simulink model "MI6FS_HE_6PhS"  (R2023a)
settings: Solver=FixedStepAuto  StartTime=0  StopTime=L  FixedStep=Ts  RelTol=1e-3
values from neighbouring files (symbols this model uses):
  A = exp(j*pi/3)    [Parameters.m]
  deg = 0    [Parameters.m]
  FV = 9.8    [Parameters.m]
  J = 0.0243    [Parameters.m]
  Lrr = [((1/3*Lm)+Llr) 1/6*Lm -1/6*Lm -1/3*Lm -1/6*Lm 1/6*Lm;        1/6*Lm ((1/3*Lm)+Llr) 1/6*Lm -1/6*Lm -1/3*Lm -1/6*Lm;        -1/6*Lm 1/6*Lm ((1/3*Lm)+Llr) 1/6*Lm -1/6*Lm -1/3*Lm;        -1/3*Lm -1/6*Lm 1/6*Lm ((1/3*Lm)+Llr) 1/6*Lm -1/6*Lm;        -1/6*Lm -1/3*Lm -1/6*Lm 1/6*Lm ((1/3*Lm)+Llr) 1/6*Lm;        1/6*Lm -1/6*Lm -1/3*Lm -1/6*Lm 1/6*Lm ((1/3*Lm)+Llr)]    [Parameters.m]
  Lrs = transpose(Lsr)    [Parameters.m]
  Lsr = [0 (pi/3) 2*(pi/3) 3*(pi/3) 4*(pi/3) 5*(pi/3);        -(pi/3) 0 (pi/3) 2*(pi/3) 3*(pi/3) 4*(pi/3);        -2*(pi/3) -(pi/3) 0 (pi/3) 2*(pi/3) 3*(pi/3);        -3*(pi/3) -2*(pi/3) -(pi/3) 0 (pi/3) 2*(pi/3);        -4*(pi/3) -3*(pi/3) -2*(pi/3) -(pi/3) 0 (pi/3);        -5*(pi/3) -4*(pi/3) -3*(pi/3) -2*(pi/3) -(pi/3) 0]    [Parameters.m]
  Lss = [((1/3*Lm)+Lls) 1/6*Lm -1/6*Lm -1/3*Lm -1/6*Lm 1/6*Lm;        1/6*Lm ((1/3*Lm)+Lls) 1/6*Lm -1/6*Lm -1/3*Lm -1/6*Lm;        -1/6*Lm 1/6*Lm ((1/3*Lm)+Lls) 1/6*Lm -1/6*Lm -1/3*Lm;        -1/3*Lm -1/6*Lm 1/6*Lm ((1/3*Lm)+Lls) 1/6*Lm -1/6*Lm;        -1/6*Lm -1/3*Lm -1/6*Lm 1/6*Lm ((1/3*Lm)+Lls) 1/6*Lm;        1/6*Lm -1/6*Lm -1/3*Lm -1/6*Lm 1/6*Lm ((1/3*Lm)+Lls)]    [Parameters.m]
  Lto = 0    [Parameters.m]
  Msr = (1/3)*Lm    (= 0.0620333333333)    [Parameters.m]
  p = 2    [Parameters.m]
  Rcore = 811    [Parameters.m]
  Rrr = Rr*eye(6,6)    [Parameters.m]
  Rss = Rs*eye(6,6)    [Parameters.m]
  Tav = 0.23    [Parameters.m]
  Ts = 1/Fs    (= 1e-05)    [Parameters.m]
  Us = sqrt(2)*180    [Parameters.m]
undefined symbols (not defined in the file or in its folder): DiscIntNeverNeededParam, j
libraries: spsFourierLib x84, spsVoltageMeasurementLib x13, spsACVoltageSourceLib x6, spsControlledCurrentSourceLib x6, spsCurrentMeasurementLib x6, spsSeriesRLCBranchLib x6, spsSequenceAnalyzerLib x6, sharedutil x5, eeRmsMeasurement x2, eeGeneralControl x1, spsSequenceAnalyzerPhasorLib x1, spsabctoAlphaBetaZeroLib x1
(part 1 of 3)
settings Model: Creator=Hugo  LastModifiedBy=HUGO
settings SolverCC: AlgebraicLoopSolver=TrustRegion
settings DataIOCC: SaveFormat=StructureWithTime  SaveTime=off
settings DebuggingCC: UnconnectedInputMsg=warning  UnconnectedOutputMsg=warning  UnconnectedLineMsg=warning  UnderSpecifiedDimensionMsg=warning
settings ModelReferenceCC: EnableRefExpFcnMdlSchedulingChecks=on
settings SFSimCC: CustomCodeUndefinedFunction=UseInterfaceOnly
settings RTWCC: DLArmComputeVersion=19.05

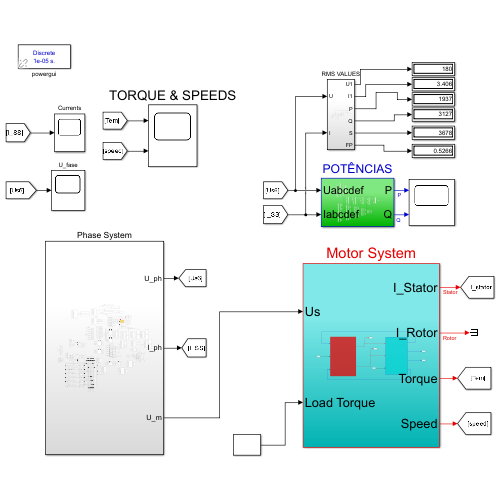
[thumbnail: Simulink's stored preview of the top-level diagram]
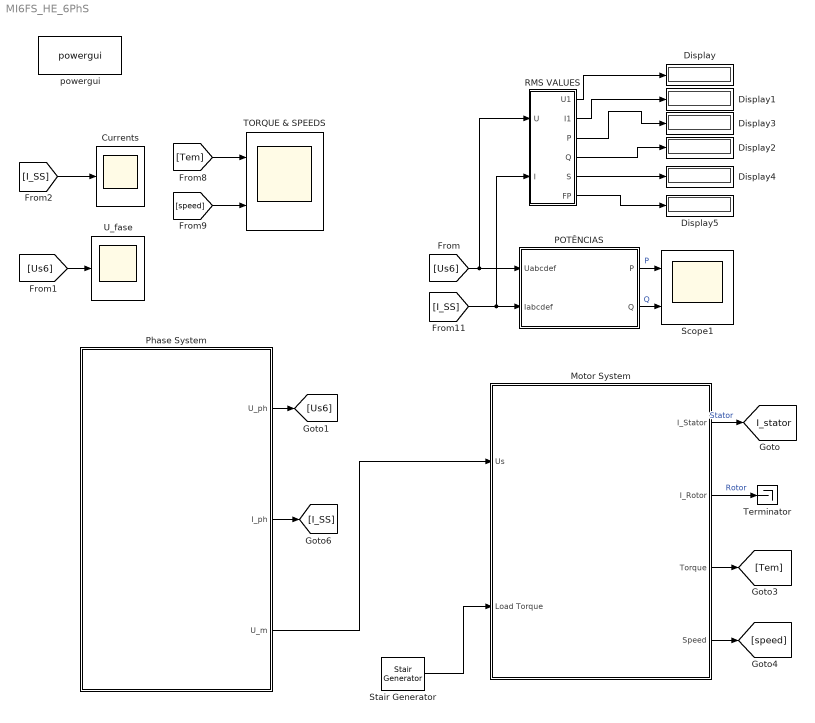
== system MI6FS_HE_6PhS ==
  Currents : Scope
  Display{,1..5} (6 alike) : Display
  Motor System : Subsystem
  POTÊNCIAS : Subsystem
  Phase System : Subsystem
  RMS VALUES : Subsystem
  Scope1 : Scope  NumInputPorts=2
  Stair Generator : spsStairGeneratorLib/Stair Generator  t=[0, 0.5]  e=[0, FV]  Ts=Ts
  TORQUE & SPEEDS : Scope  NumInputPorts=2
  Terminator : Terminator
  U_fase : Scope
  powergui : spspowerguiLib/powergui  Priority=1  SimulationMode=Discrete  SampleTime=Ts  frequency=60  Iterations=50  frequencyindice=50  Pbase=100e6  ErrMax=1e-4  UnitsV=kV  UnitsW=MW  buscounter=0  FunctionMessages=off  echomessages=off  EnableUseOfTLC=off  CurrentSourceSwitches=off  DisableSnubberDevices=off  DisableRonSwitches=off  DisableVfSwitches=off  DisplayEquations=off  AutomaticDiscreteSolvers=off  SolverType=Tustin/Backward Euler (TBE)  Interpol=off  ExternalGateDelay=off  methode=off  Ts=100  x0status=blocks  SPID=on  SwTol=0  HookPort=off  NonlinearTolerance=0  nMaxIteration=15  ContinueOnMaxIteration=off  RestoreLinks=warning  ResistiveCurrentMeasurement=off  Frange=[0:2:500]  Ylog=off  Xlog=on  ShowGrid=off  save=off  variable=ZData  structure=0  ZoomFFT=off  StartTime=0.0  cycles=1  DisplayStyle=1  fundamental=60  FreqAxis=off  MaxFrequency=1000  frequencyindicesteady=1  RmsSteady=1  display=off
  tag scope: I_stator=global
  wires:
  POTÊNCIAS/1(P) -> Scope1/1  "P"
  POTÊNCIAS/2(Q) -> Scope1/2  "Q"
  Motor System/1(I_Stator) -> [I_stator]  "Stator"
  [I_SS] -> POTÊNCIAS/2(Iabcdef), RMS VALUES/2(I)
  Motor System/2(I_Rotor) -> Terminator/1  "Rotor"
  Motor System/3(Torque) -> [Tem]
  Motor System/4(Speed) -> [speed]
  RMS VALUES/1(U1) -> Display/1
  RMS VALUES/2(I1) -> Display1/1
  RMS VALUES/4(Q) -> Display2/1
  RMS VALUES/3(P) -> Display3/1
  RMS VALUES/5(S) -> Display4/1
  RMS VALUES/6(FP) -> Display5/1
  [Us6] -> POTÊNCIAS/1(Uabcdef), RMS VALUES/1(U)
  [Tem] -> TORQUE & SPEEDS/1
  [speed] -> TORQUE & SPEEDS/2
  Phase System/3(U_m) -> Motor System/1(Us)
  Stair Generator/1 -> Motor System/2(Load Torque)
  Phase System/1(U_ph) -> [Us6]
  Phase System/2(I_ph) -> [I_SS]
  [I_SS] -> Currents/1
  [Us6] -> U_fase/1

== system MI6FS_HE_6PhS/Motor System ==
  Us : Inport
  Load Torque : Inport  Port=2
  MECHANICAL SYSTEM : Subsystem
  "MOTOR SYSTEM EQUATIONS " : Subsystem
  I_Stator : Outport  VectorParamsAs1DForOutWhenUnconnected=off
  I_Rotor : Outport  Port=2  VectorParamsAs1DForOutWhenUnconnected=off
  Torque : Outport  Port=3  VectorParamsAs1DForOutWhenUnconnected=off
  Speed : Outport  Port=4  VectorParamsAs1DForOutWhenUnconnected=off
  wires:
  "MOTOR SYSTEM EQUATIONS "/1(I_stator) -> I_Stator/1, MECHANICAL SYSTEM/1(I_s)
  Load Torque/1 -> MECHANICAL SYSTEM/3(TLoad)
  "MOTOR SYSTEM EQUATIONS "/2("I_rotor ") -> MECHANICAL SYSTEM/2(I_r), I_Rotor/1
  Us/1 -> "MOTOR SYSTEM EQUATIONS "/2(Us)
  MECHANICAL SYSTEM/4("Teta_R [rad] ") -> "MOTOR SYSTEM EQUATIONS "/3(Teta_R)
  MECHANICAL SYSTEM/1(We [rads/s]) -> "MOTOR SYSTEM EQUATIONS "/1(We)
  MECHANICAL SYSTEM/2(Tem [Nm]) -> Torque/1
  MECHANICAL SYSTEM/3(n [rpm]) -> Speed/1

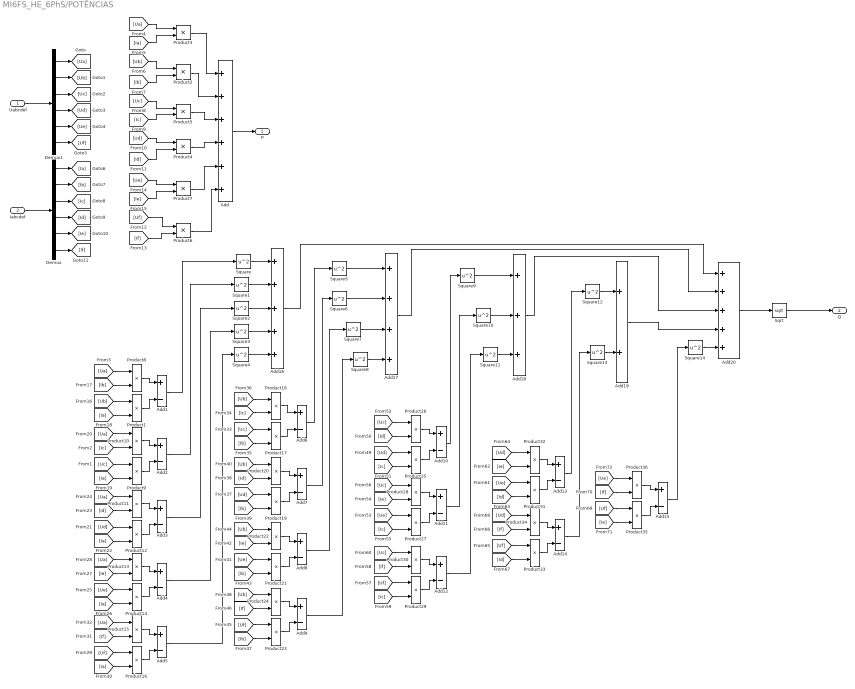
== system MI6FS_HE_6PhS/POTÊNCIAS ==
  Uabcdef : Inport
  Iabcdef : Inport  Port=2
  Add : Sum  Inputs=6
  Add{1..15} (15 alike) : Sum  Inputs=+-
  Add16 : Sum  Inputs=+++++
  Add17 : Sum  Inputs=++++
  Add18 : Sum  Inputs=+++
  Add19 : Sum
  Add20 : Sum  Inputs=5
  Demux : Demux  Outputs=6
  Demux1 : Demux  Outputs=6
  Product{1..36} (36 alike) : Product
  Sqrt : Sqrt
  Square{,1..14} (15 alike) : Math  Operator=square  SignedPower=on
  P : Outport  VectorParamsAs1DForOutWhenUnconnected=off
  Q : Outport  Port=2  VectorParamsAs1DForOutWhenUnconnected=off
  wires:
  Iabcdef/1 -> Demux/1
  Uabcdef/1 -> Demux1/1
  Demux1/1 -> [Ua]
  Demux1/2 -> [Ub]
  Demux1/3 -> [Uc]
  Demux1/4 -> [Ud]
  Demux1/5 -> [Ue]
  Demux1/6 -> [Uf]
  Demux/1 -> [Ia]
  Demux/2 -> [Ib]
  Demux/3 -> [Ic]
  Demux/6 -> [If]
  Demux/4 -> [Id]
  Demux/5 -> [Ie]
  [Ud] -> Product4/1
  [Id] -> Product4/2
  [Ue] -> Product7/1
  [Ie] -> Product7/2
  [Uf] -> Product6/1
  Product2/1 -> Add/2
  Product5/1 -> Add/3
  Product4/1 -> Add/4
  Product7/1 -> Add/5
  Product6/1 -> Add/6
  Product3/1 -> Add/1
  Add/1 -> P/1
  [Ic] -> Product5/2
  [Uc] -> Product5/1
  [Ie] -> Product28/2
  Product17/1 -> Add6/2
  [Id] -> Product33/2
  [If] -> Product30/2
  [Ic] -> Product25/2
  Product32/1 -> Add13/1
  Product30/1 -> Add12/1
  [Ic] -> Product29/2
  [Ia] -> Product9/2
  Product8/1 -> Add1/1
  [Uf] -> Product29/1
  Product15/1 -> Add5/1
  [Id] -> Product26/2
  Product19/1 -> Add7/2
  [Ue] -> Product27/1
  [Ub] -> Product24/1
  [Ud] -> Product25/1
  Product24/1 -> Add9/1
  [Ib] -> Product23/2
  [Uc] -> Product28/1
  Product27/1 -> Add11/2
  Product25/1 -> Add10/2
  [Ib] -> Product21/2
  [Ua] -> Product8/1
  [Ub] -> Product22/1
  [Ue] -> Product21/1
  [Ie] -> Product22/2
  [Uc] -> Product17/1
  Product20/1 -> Add7/1
  Product21/1 -> Add8/2
  [Id] -> Product20/2
  Product18/1 -> Add6/1
  [Ic] -> Product18/2
  Product16/1 -> Add5/2
  [Ua] -> Product10/1
  [Ud] -> Product12/1
  [Ub] -> Product18/1
  [Ib] -> Product8/2
  [If] -> Product15/2
  [Id] -> Product11/2
  Product14/1 -> Add4/2
  [Ue] -> Product14/1
  Product13/1 -> Add4/1
  Product10/1 -> Add2/1
  [Ua] -> Product11/1
  Product11/1 -> Add3/1
  [Ud] -> Product19/1
  [Ub] -> Product1/1
  Add17/1 -> Add20/2
  [Ib] -> Product19/2
  Add6/1 -> Square5/1
  Add15/1 -> Square14/1
  [Uc] -> Product26/1
  Add19/1 -> Add20/4
  Add16/1 -> Add20/1
  Add7/1 -> Square6/1
  [Ia] -> Product16/2
  Product23/1 -> Add9/2
  [Id] -> Product31/2
  [Ie] -> Product13/2
  Add10/1 -> Square9/1
  [Ie] -> Product32/2
  [Ia] -> Product12/2
  Product29/1 -> Add12/2
  [Ue] -> Product31/1
  Product35/1 -> Add15/2
  Product12/1 -> Add3/2
  [Ia] -> Product14/2
  [Ub] -> Product20/1
  Product28/1 -> Add11/1
  Add12/1 -> Square11/1
  Add14/1 -> Square13/1
  Add3/1 -> Square2/1
  Add11/1 -> Square10/1
  [Ic] -> Product10/2
  Add9/1 -> Square8/1
  [Ib] -> Product17/2
  Add13/1 -> Square12/1
  Add18/1 -> Add20/3
  [Ua] -> Product15/1
  Add1/1 -> Square/1
  [Ua] -> Product13/1
  Product36/1 -> Add15/1
  Add4/1 -> Square3/1
  Add2/1 -> Square1/1
  [If] -> Product36/2
  Add5/1 -> Square4/1
  [Uf] -> Product33/1
  [If] -> Product24/2
  Product9/1 -> Add2/2
  Product1/1 -> Add1/2
  [Uc] -> Product9/1
  Add8/1 -> Square7/1
  [Uf] -> Product23/1
  Product22/1 -> Add8/1
  [Uc] -> Product30/1
  Product26/1 -> Add10/1
  [Ud] -> Product32/1
  [Ia] -> Product1/2
  [Uf] -> Product16/1
  Product33/1 -> Add14/2
  [Uf] -> Product35/1
  Product31/1 -> Add13/2
  [Ie] -> Product35/2
  [Ue] -> Product36/1
  [If] -> Product34/2
  [Ic] -> Product27/2
  Product34/1 -> Add14/1
  [Ud] -> Product34/1
  [Ua] -> Product3/1
  [Ub] -> Product2/1
  [If] -> Product6/2
  Sqrt/1 -> Q/1
  Square/1 -> Add16/1
  Square1/1 -> Add16/2
  Square2/1 -> Add16/3
  Square3/1 -> Add16/4
  Square4/1 -> Add16/5
  Square5/1 -> Add17/1
  Square6/1 -> Add17/2
  Square7/1 -> Add17/3
  Square8/1 -> Add17/4
  Square9/1 -> Add18/1
  Square10/1 -> Add18/2
  Square11/1 -> Add18/3
  Square12/1 -> Add19/1
  Square13/1 -> Add19/2
  Square14/1 -> Add20/5
  Add20/1 -> Sqrt/1
  [Ia] -> Product3/2
  [Ib] -> Product2/2

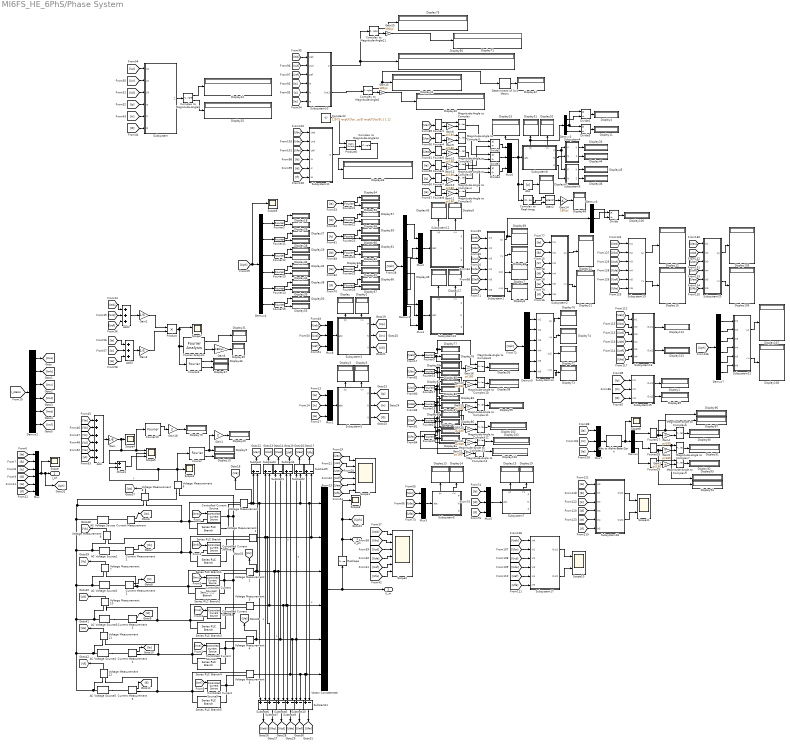
== system MI6FS_HE_6PhS/Phase System ==
  AC Voltage Source : spsACVoltageSourceLib/AC Voltage Source  Amplitude=Us  Phase=deg  Frequency=50  SampleTime=Ts  Measurements=None  BusType=swing  Pref=10e3  Qref=0  Qmin=-inf  Qmax=+inf
  AC Voltage Source1 : spsACVoltageSourceLib/AC Voltage Source  Amplitude=Us  Phase=-60  Frequency=50  SampleTime=Ts  Measurements=None  BusType=swing  Pref=10e3  Qref=0  Qmin=-inf  Qmax=+inf
  AC Voltage Source2 : spsACVoltageSourceLib/AC Voltage Source  Amplitude=Us  Phase=-120  Frequency=50  SampleTime=Ts  Measurements=None  BusType=swing  Pref=10e3  Qref=0  Qmin=-inf  Qmax=+inf
  AC Voltage Source3 : spsACVoltageSourceLib/AC Voltage Source  Amplitude=Us  Phase=-180  Frequency=50  SampleTime=Ts  Measurements=None  BusType=swing  Pref=10e3  Qref=0  Qmin=-inf  Qmax=+inf
  AC Voltage Source4 : spsACVoltageSourceLib/AC Voltage Source  Amplitude=Us  Phase=-240  Frequency=50  SampleTime=Ts  Measurements=None  BusType=swing  Pref=10e3  Qref=0  Qmin=-inf  Qmax=+inf
  AC Voltage Source5 : spsACVoltageSourceLib/AC Voltage Source  Amplitude=Us  Phase=-300  Frequency=50  SampleTime=Ts  Measurements=None  BusType=swing  Pref=10e3  Qref=0  Qmin=-inf  Qmax=+inf
  Abs : Abs  SaturateOnIntegerOverflow=off
  Add : Sum  Inputs=6
  Add2 : Sum  Inputs=3
  Add3 : Sum  Inputs=3
  Atan2 : Trigonometry  Operator=atan2
  Complex to Magnitude-Angle{2..3,14,21} (4 alike) : ComplexToMagnitudeAngle
  Complex to Real-Imag : ComplexToRealImag
  Constant2 : Constant  Value=1/3*[1 exp(j*2*pi/3) exp(j*4*pi/3); 1 exp(j*4*pi/3) exp(j*2*pi/3);1 1 1]
  Controlled Current Source{,1..5} (6 alike) : spsControlledCurrentSourceLib/Controlled Current Source  Initialize=off  Source_Type=DC  Amplitude=0  Phase=0  Frequency=0  Measurements=None
  Current Measurement{,1..5} (6 alike) : spsCurrentMeasurementLib/Current Measurement  PhasorSimulation=off  OutputType=Complex  PSBequivalent=0
  Demux : Demux  Outputs=3
  Demux{1..2,4..5,7} (5 alike) : Demux  Outputs=6
  Demux3 : Demux  Outputs=3
  Demux6 : Demux  Outputs=3
  Determinant of 3x3 Matrix : sharedutil/Determinant of 3x3 Matrix  aMode=aMode
  Display{,1..108,112} (110 alike) : Display
  Divide{,1..5} (6 alike) : Product  Inputs=*/
  Fourier : spsFourierLib/Fourier  Freq=50  n=1  InInit=[0, 0]  Ts=0
  Fourier Analysis : eeGeneralControl/Fourier Analysis  f=50  n="[0  2]"  M0=0  Ph0=0  BufferSize=8192  Ts=Ts
  Fourier{1..2,4..9,11..29} (27 alike) : spsFourierLib/Fourier  Freq=50  n=1  InInit=[0, 0]  Ts=Ts
  Fourier10 : spsFourierLib/Fourier  Freq=50  n=1  InInit=[0, 0]  Ts=0
  Fourier3 : spsFourierLib/Fourier  Freq=50  n=0  InInit=[0, 0]  Ts=0
  Gain : Gain  Gain=1/6
  Gain1 : Gain  Gain=2
  Gain{4..5,7..13,16..17,19..22} (15 alike) : Gain  Gain=pi/180
  Gain{6,14..15,25} (4 alike) : Gain  Gain=180/pi
  Gain18 : Gain  Gain=2
  Gain2 : Gain  Gain=1/3
  Gain3 : Gain  Gain=1/3
  Magnitude-Angle to Complex{,1..14} (15 alike) : MagnitudeAngleToComplex
  Minus1 : Sum  Inputs=+-
  Mux : Mux  Inputs=6
  Mux{1..8} (8 alike) : Mux  Inputs=3
  Product : Product
  Product6 : Product  Multiplication=Matrix(*)
  Reshape : Reshape  OutputDimensionality=Customize  OutputDimensions=6
  Scope{,3..4,6,8..9} (6 alike) : Scope
  Scope1 : Scope  NumInputPorts=6
  Scope10 : Scope  NumInputPorts=2
  Scope11 : Scope  NumInputPorts=2
  Scope2 : Scope  NumInputPorts=6
  Scope5 : Scope  NumInputPorts=3
  Scope7 : Scope  NumInputPorts=2
  Series RLC Branch{,1..5} (6 alike) : spsSeriesRLCBranchLib/Series RLC Branch  LConnTagsString=__new0  RConnTagsString=__new0  BranchType=R  Resistance=Rcore  Inductance=1e-3  SetiL0=off  InitialCurrent=0  Capacitance=1e-6  Setx0=off  InitialVoltage=0  Measurements=None
  Subsystem : Subsystem
  Subsystem1 : Subsystem
  Subsystem10 : Subsystem
  Subsystem11 : Subsystem
  Subsystem12 : Subsystem
      settings: PortSchema="{\"entries\":[{\"content\":{\"sides\":[{\"content\":{\"connectorIds\":[\"In1\"]},\"type\":\"ConnectorPlacement.EquallySpacedRectSide\",\"uuid\":\"08bafebd-79cb-449b-bcfd-66ce530336a5\"},{\"content\":{\"connectorIds\":[\"Out1\",\"Out2\",\"Out3\"],\"side\":\"RIGHT\"},\"type\":\"ConnectorPlacement.EquallySpacedRectSide\",\"uuid\":\"938c76d8-1425-4a37-80e8-b201e4c6d43d\"},{\"content\":{\"connectorIds\":[\"Out4\",\"Out5\"],\"side\":\"TOP\"},\"type\":\"ConnectorPlacement.EquallySpacedRectSide\",\"uuid\":\"53fbc516-6cef-40b0-811b-19f23fab8c53\"}]},\"type\":\"ConnectorPlacement.EquallySpacedConnector\",\"uuid\":\"c6349fbf-f101-45a6-bcbc-b95cb31e8510\"}],\"packageUris\":[\"http://schema.mathworks.com/mf0/Connector/R2020b\"],\"version\":\"1.0\"}"
  Subsystem13 : Subsystem
      settings: PortSchema="{\"entries\":[{\"content\":{\"sides\":[{\"content\":{\"connectorIds\":[\"In1\"]},\"type\":\"ConnectorPlacement.EquallySpacedRectSide\",\"uuid\":\"08bafebd-79cb-449b-bcfd-66ce530336a5\"},{\"content\":{\"connectorIds\":[\"Out1\",\"Out2\",\"Out3\"],\"side\":\"RIGHT\"},\"type\":\"ConnectorPlacement.EquallySpacedRectSide\",\"uuid\":\"938c76d8-1425-4a37-80e8-b201e4c6d43d\"},{\"content\":{\"connectorIds\":[\"Out4\",\"Out5\"],\"side\":\"TOP\"},\"type\":\"ConnectorPlacement.EquallySpacedRectSide\",\"uuid\":\"53fbc516-6cef-40b0-811b-19f23fab8c53\"}]},\"type\":\"ConnectorPlacement.EquallySpacedConnector\",\"uuid\":\"c6349fbf-f101-45a6-bcbc-b95cb31e8510\"}],\"packageUris\":[\"http://schema.mathworks.com/mf0/Connector/R2020b\"],\"version\":\"1.0\"}"
  Subsystem14 : Subsystem
  Subsystem15 : Subsystem
  Subsystem16 : Subsystem
  Subsystem17 : Subsystem
  Subsystem18 : Subsystem
  Subsystem19 : Subsystem
  Subsystem2 : Subsystem
  Subsystem20 : Subsystem
  Subsystem21 : Subsystem
  Subsystem3 : Subsystem
      settings: PortSchema="{\"entries\":[{\"content\":{\"sides\":[{\"content\":{\"connectorIds\":[\"In1\"]},\"type\":\"ConnectorPlacement.EquallySpacedRectSide\",\"uuid\":\"08bafebd-79cb-449b-bcfd-66ce530336a5\"},{\"content\":{\"connectorIds\":[\"Out1\",\"Out2\",\"Out3\"],\"side\":\"RIGHT\"},\"type\":\"ConnectorPlacement.EquallySpacedRectSide\",\"uuid\":\"938c76d8-1425-4a37-80e8-b201e4c6d43d\"},{\"content\":{\"connectorIds\":[\"Out4\",\"Out5\"],\"side\":\"TOP\"},\"type\":\"ConnectorPlacement.EquallySpacedRectSide\",\"uuid\":\"53fbc516-6cef-40b0-811b-19f23fab8c53\"}]},\"type\":\"ConnectorPlacement.EquallySpacedConnector\",\"uuid\":\"c6349fbf-f101-45a6-bcbc-b95cb31e8510\"}],\"packageUris\":[\"http://schema.mathworks.com/mf0/Connector/R2020b\"],\"version\":\"1.0\"}"
  Subsystem4 : Subsystem
  Subsystem5 : Subsystem
      settings: PortSchema="{\"entries\":[{\"content\":{\"sides\":[{\"content\":{\"connectorIds\":[\"In1\"]},\"type\":\"ConnectorPlacement.EquallySpacedRectSide\",\"uuid\":\"08bafebd-79cb-449b-bcfd-66ce530336a5\"},{\"content\":{\"connectorIds\":[\"Out1\",\"Out2\",\"Out3\"],\"side\":\"RIGHT\"},\"type\":\"ConnectorPlacement.EquallySpacedRectSide\",\"uuid\":\"938c76d8-1425-4a37-80e8-b201e4c6d43d\"},{\"content\":{\"connectorIds\":[\"Out4\",\"Out5\"],\"side\":\"TOP\"},\"type\":\"ConnectorPlacement.EquallySpacedRectSide\",\"uuid\":\"53fbc516-6cef-40b0-811b-19f23fab8c53\"}]},\"type\":\"ConnectorPlacement.EquallySpacedConnector\",\"uuid\":\"c6349fbf-f101-45a6-bcbc-b95cb31e8510\"}],\"packageUris\":[\"http://schema.mathworks.com/mf0/Connector/R2020b\"],\"version\":\"1.0\"}"
  Subsystem6 : Subsystem
      settings: PortSchema="{\"entries\":[{\"content\":{\"sides\":[{\"content\":{\"connectorIds\":[\"In1\"]},\"type\":\"ConnectorPlacement.EquallySpacedRectSide\",\"uuid\":\"08bafebd-79cb-449b-bcfd-66ce530336a5\"},{\"content\":{\"connectorIds\":[\"Out1\",\"Out2\",\"Out3\"],\"side\":\"RIGHT\"},\"type\":\"ConnectorPlacement.EquallySpacedRectSide\",\"uuid\":\"938c76d8-1425-4a37-80e8-b201e4c6d43d\"},{\"content\":{\"connectorIds\":[\"Out4\",\"Out5\"],\"side\":\"TOP\"},\"type\":\"ConnectorPlacement.EquallySpacedRectSide\",\"uuid\":\"53fbc516-6cef-40b0-811b-19f23fab8c53\"}]},\"type\":\"ConnectorPlacement.EquallySpacedConnector\",\"uuid\":\"c6349fbf-f101-45a6-bcbc-b95cb31e8510\"}],\"packageUris\":[\"http://schema.mathworks.com/mf0/Connector/R2020b\"],\"version\":\"1.0\"}"
  Subsystem7 : Subsystem
      settings: PortSchema="{\"entries\":[{\"content\":{\"sides\":[{\"content\":{\"connectorIds\":[\"In1\"]},\"type\":\"ConnectorPlacement.EquallySpacedRectSide\",\"uuid\":\"08bafebd-79cb-449b-bcfd-66ce530336a5\"},{\"content\":{\"connectorIds\":[\"Out1\",\"Out2\",\"Out3\"],\"side\":\"RIGHT\"},\"type\":\"ConnectorPlacement.EquallySpacedRectSide\",\"uuid\":\"938c76d8-1425-4a37-80e8-b201e4c6d43d\"},{\"content\":{\"connectorIds\":[\"Out4\",\"Out5\"],\"side\":\"TOP\"},\"type\":\"ConnectorPlacement.EquallySpacedRectSide\",\"uuid\":\"53fbc516-6cef-40b0-811b-19f23fab8c53\"}]},\"type\":\"ConnectorPlacement.EquallySpacedConnector\",\"uuid\":\"c6349fbf-f101-45a6-bcbc-b95cb31e8510\"}],\"packageUris\":[\"http://schema.mathworks.com/mf0/Connector/R2020b\"],\"version\":\"1.0\"}"
  Subsystem8 : Subsystem
      settings: PortSchema="{\"entries\":[{\"content\":{\"sides\":[{\"content\":{\"connectorIds\":[\"In1\"]},\"type\":\"ConnectorPlacement.EquallySpacedRectSide\",\"uuid\":\"08bafebd-79cb-449b-bcfd-66ce530336a5\"},{\"content\":{\"connectorIds\":[\"Out1\",\"Out2\",\"Out3\"],\"side\":\"RIGHT\"},\"type\":\"ConnectorPlacement.EquallySpacedRectSide\",\"uuid\":\"938c76d8-1425-4a37-80e8-b201e4c6d43d\"},{\"content\":{\"connectorIds\":[\"Out4\",\"Out5\"],\"side\":\"TOP\"},\"type\":\"ConnectorPlacement.EquallySpacedRectSide\",\"uuid\":\"53fbc516-6cef-40b0-811b-19f23fab8c53\"}]},\"type\":\"ConnectorPlacement.EquallySpacedConnector\",\"uuid\":\"c6349fbf-f101-45a6-bcbc-b95cb31e8510\"}],\"packageUris\":[\"http://schema.mathworks.com/mf0/Connector/R2020b\"],\"version\":\"1.0\"}"
  Subsystem9 : Subsystem
  Subtract{,1..11} (12 alike) : Sum  Inputs=+-
  Vector Concatenate : Concatenate  NumInputs=6  Mode=Multidimensional array
  Voltage Measurement{,1..12} (13 alike) : spsVoltageMeasurementLib/Voltage Measurement  PhasorSimulation=off  OutputType=Complex  PSBequivalent=0
  abc to Alpha-Beta-Zero : spsabctoAlphaBetaZeroLib/abc to Alpha-Beta-Zero
  U_ph : Outport
  I_ph : Outport  Port=2
  U_m : Outport  Port=3
  wires:
  Voltage Measurement3/1 -> Subtract3/2, Subtract8/2, Subtract4/1, Subtract9/1, Vector Concatenate/4  "d"
  Voltage Measurement4/1 -> Subtract1/2, Subtract9/2, Subtract10/1, Subtract2/1, Vector Concatenate/5, [Ue]  "e"
  Voltage Measurement2/1 -> Subtract/2, Subtract7/2, Subtract8/1, Vector Concatenate/3, Subtract1/1, [Uc]  "c"
  Voltage Measurement/1 -> [Ua], Subtract2/2, Vector Concatenate/1, Subtract11/2, Subtract6/1, Subtract/1  "a"
  Voltage Measurement5/1 -> Subtract4/2, Subtract10/2, Subtract11/1, Vector Concatenate/6, Subtract5/1
  Voltage Measurement1/1 -> Subtract6/2, Subtract3/1, Subtract7/1, Subtract5/2, Vector Concatenate/2  "b"
  Vector Concatenate/1 -> U_m/1, Reshape/1
  [I_stator] -> Demux2/1
  Demux2/1 -> [Ima]
  Demux2/2 -> [Imb]
  Demux2/3 -> [Imc]
  Demux2/4 -> [Imd]
  Demux2/5 -> [Ime]
  Demux2/6 -> [Imf]
  [Ima] -> Controlled Current Source/1
  [Imb] -> Controlled Current Source1/1
  [Imc] -> Controlled Current Source2/1
  [Imd] -> Controlled Current Source3/1
  [Ime] -> Controlled Current Source4/1
  [Imf] -> Controlled Current Source5/1
  Current Measurement/1 -> [Ia]
  Current Measurement1/1 -> [Ib]
  Current Measurement2/1 -> [Ic]
  Current Measurement3/1 -> [Id]
  Current Measurement4/1 -> [Ie]
  Current Measurement5/1 -> [If]
  [Ia] -> Mux/1
  [Ib] -> Mux/2
  [Ic] -> Mux/3
  [Id] -> Mux/4
  [Ie] -> Mux/5
  [If] -> Mux/6
  Mux/1 -> Scope/1, [Iph], I_ph/1
  Subtract/1 -> [Uac]
  Subtract3/1 -> [Ubd]
  Subtract1/1 -> [Uce]
  Subtract4/1 -> [Udf]
  Subtract2/1 -> [Uea]
  Subtract5/1 -> [Ufb]
  [Uac] -> Scope1/1
  [Ubd] -> Scope1/2
  [Uce] -> Scope1/3
  [Udf] -> Scope1/4
  [Uea] -> Scope1/5
  [Ufb] -> Scope1/6
  Subtract6/1 -> [Uab]
  Subtract7/1 -> [Ubc]
  Subtract8/1 -> [Ucd]
  Subtract9/1 -> [Ude]
  Subtract10/1 -> [Uef]
  Subtract11/1 -> [Ufa]
  [Uab] -> Scope2/1
  [Ubc] -> Scope2/2
  [Ucd] -> Scope2/3
  [Ude] -> Scope2/4
  [Uef] -> Scope2/5
  [Ufa] -> Scope2/6
  [Uab] -> Mux8/1
  [Ucd] -> Mux8/2
  [Uef] -> Mux8/3
  [Ie] -> Mux1/3
  [Ic] -> Mux1/2
  [Ia] -> Mux1/1
  Mux8/1 -> Subsystem3/1(abc)
  Subsystem3/5(<u) -> Display2/1
  Mux1/1 -> Subsystem5/1(abc)
  Subsystem5/5(<u) -> Display5/1
  Subsystem5/1(P) -> [Ip]
  Subsystem3/2(N) -> [Un]
  Subsystem3/1(P) -> [Up]
  Subsystem5/2(N) -> [In]
  Subsystem5/3(0) -> [I0]
  Voltage Measurement6/1 -> Scope3/1, Fourier/1, Minus1/2, Scope5/2  "f"
  [Va] -> Add/1
  [Vb] -> Add/2
  [Vc] -> Add/3
  [Vd] -> Add/4
  [Ve] -> Add/5
  [Vf] -> Add/6
  Add/1 -> Gain/1
  Voltage Measurement8/1 -> [Va]
  Voltage Measurement9/1 -> [Vb]
  Voltage Measurement7/1 -> [Vc]
  Voltage Measurement10/1 -> [Vd]
  Voltage Measurement11/1 -> [Ve]
  Voltage Measurement12/1 -> [Vf]
  Gain/1 -> Scope4/1, Fourier10/1, Scope5/1, Minus1/1
  Subsystem5/4(|u|) -> Display3/1
  Subsystem3/4(|u|) -> Display/1
  Minus1/1 -> Scope5/3
  Fourier/1 -> Gain1/1, Display9/1
  Fourier/2 -> Display10/1
  [Ude] -> Mux3/2
  [Ubc] -> Mux3/1
  [Ufa] -> Mux3/3
  Subsystem6/4(|u|) -> Display13/1
  Mux3/1 -> Subsystem6/1(abc)
  Subsystem6/5(<u) -> Display14/1
  [Id] -> Mux5/2
  [Ib] -> Mux5/1
  [If] -> Mux5/3
  Subsystem7/4(|u|) -> Display15/1
  Subsystem7/5(<u) -> Display19/1
  Gain1/1 -> Display20/1
  [Uab] -> Add2/1
  [Ucd] -> Add2/2
  [Uef] -> Add2/3
  [Ia] -> Add3/1
  [Ic] -> Add3/2
  [Ie] -> Add3/3
  Add2/1 -> Gain2/1
  Add3/1 -> Gain3/1
  Gain2/1 -> Product/1
  Gain3/1 -> Product/2
  Product/1 -> Fourier3/1, Fourier Analysis/1, Scope7/1
  Mux6/1 -> Subsystem8/1(abc), Display23/1, Complex to Real-Imag/1, Abs/1
  Magnitude-Angle to Complex5/1 -> Divide4/2
  Gain8/1 -> Magnitude-Angle to Complex/2
  Fourier1/2 -> Gain8/1
  Divide4/1 -> Mux6/3
  Divide3/1 -> Mux6/2
  Divide2/1 -> Mux6/1
  Gain12/1 -> Magnitude-Angle to Complex2/2
  Fourier5/2 -> Gain12/1
  Fourier5/1 -> Magnitude-Angle to Complex2/1
  Subsystem8/5(<u) -> Display52/1
  Magnitude-Angle to Complex1/1 -> Divide3/1
  Magnitude-Angle to Complex3/1 -> Divide2/2
  Fourier7/2 -> Gain10/1
  Fourier6/2 -> Gain13/1
  Gain13/1 -> Magnitude-Angle to Complex3/2
  Gain10/1 -> Magnitude-Angle to Complex4/2
  Fourier7/1 -> Magnitude-Angle to Complex4/1
  Fourier8/1 -> Magnitude-Angle to Complex5/1
  [Uea] -> Fourier5/1
  Subsystem8/4(|u|) -> Demux3/1, Display51/1
  [Uac] -> Fourier1/1
  [Ie] -> Fourier8/1
  Fourier1/1 -> Magnitude-Angle to Complex/1
  Gain9/1 -> Magnitude-Angle to Complex1/2
  Fourier6/1 -> Magnitude-Angle to Complex3/1
  Magnitude-Angle to Complex4/1 -> Divide3/2
  [Ia] -> Fourier6/1
  Magnitude-Angle to Complex2/1 -> Divide4/1
  Fourier4/1 -> Magnitude-Angle to Complex1/1
  [Ic] -> Fourier7/1
  [Uce] -> Fourier4/1
  Fourier4/2 -> Gain9/1
  Magnitude-Angle to Complex/1 -> Divide2/1
  Gain11/1 -> Magnitude-Angle to Complex5/2
  Fourier8/2 -> Gain11/1
  Subsystem4/1(K) -> Display33/1
  Subsystem4/2(phase) -> Display44/1
  Subsystem8/1(P) -> Subsystem4/1(P), Subsystem9/1(P)
  Subsystem8/2(N) -> Subsystem4/2(N)
  Subsystem9/1(K) -> Display45/1
  Subsystem8/3(0) -> Subsystem9/2(N)
  Subsystem9/2(phase) -> Display46/1
  Abs/1 -> Display47/1
  Complex to Real-Imag/2 -> Atan2/1
  Complex to Real-Imag/1 -> Atan2/2
  Atan2/1 -> Gain14/1
  Gain14/1 -> Display48/1
  Mux5/1 -> Subsystem7/1(abc)
  [Uab] -> Subsystem10/1(Uab)
  [Ucd] -> Subsystem10/2(Ucd)
  [Uef] -> Subsystem10/3(Uef)
  [Ia] -> Subsystem10/4(Ia)
  [Ic] -> Subsystem10/5(Ic)
  [Ie] -> Subsystem10/6(Ie)
  Complex to Magnitude-Angle21/1 -> Display75/1
  Complex to Magnitude-Angle21/2 -> Gain25/1
  Gain25/1 -> Display71/1
  [Ude] -> Subsystem11/2(Ucd)
  [Ib] -> Subsystem11/4(Ia)
  [If] -> Subsystem11/6(Ie)
  [Id] -> Subsystem11/5(Ic)
  [Ufa] -> Subsystem11/3(Uef)
  [Ubc] -> Subsystem11/1(Uab)
  Subsystem11/1(Z) -> Product6/2
  Constant2/1 -> Product6/1
  Product6/1 -> Complex to Magnitude-Angle14/1
  Complex to Magnitude-Angle14/1 -> Display63/1
  Subsystem10/1(Z) -> Complex to Magnitude-Angle21/1, Display56/1
  Gain18/1 -> Display70/1
  Fourier10/1 -> Gain18/1
  Subsystem/1(Z) -> Complex to Magnitude-Angle3/1
  [Up] -> Subsystem/1(Up)
  [I0] -> Subsystem/6(I0)
  Complex to Magnitude-Angle3/2 -> Display25/1
  [In] -> Subsystem/5(In)
  [U0] -> Subsystem/3(U0)
  Complex to Magnitude-Angle3/1 -> Display24/1
  [Ip] -> Subsystem/4(Ip)
  [Un] -> Subsystem/2(Un)
  Demux3/1 -> Divide1/2
  Divide1/1 -> Display4/1
  Divide5/1 -> Display11/1
  Subsystem3/3(0) -> [U0]
  Fourier Analysis/1 -> Display31/1
  Fourier Analysis/2 -> Gain6/1
  Fourier3/1 -> Display36/1
  Fourier3/2 -> Display37/1
  Gain6/1 -> Display35/1
  Subsystem10/2(Out1) -> Complex to Magnitude-Angle2/1
  Gain15/1 -> Display40/1
  Complex to Magnitude-Angle2/2 -> Gain15/1
  Complex to Magnitude-Angle2/1 -> Determinant of 3x3 Matrix/1, Display41/1
  Determinant of 3x3 Matrix/1 -> Display42/1
  Demux3/2 -> Divide5/1, Divide1/1
  Demux3/3 -> Divide5/2
  Reshape/1 -> Scope6/1, [Uph], U_ph/1
  Demux1/4 -> Mux4/2
  Demux1/6 -> Mux4/3
  Demux1/2 -> Mux4/1
  [Uph] -> Demux1/1
  Demux1/3 -> Mux2/2
  Mux4/1 -> Subsystem13/1(abc)
  Demux1/1 -> Mux2/1
  Subsystem13/5(<u) -> Display17/1
  Subsystem13/4(|u|) -> Display49/1
  Mux2/1 -> Subsystem12/1(abc)
  Demux1/5 -> Mux2/3
  Subsystem12/4(|u|) -> Display43/1
  Subsystem12/5(<u) -> Display6/1
  Fourier12/1 -> Display29/1
  Fourier15/1 -> Display50/1
  Fourier2/2 -> Display26/1
  Demux4/5 -> Fourier14/1
  Fourier2/1 -> Display18/1
  Fourier11/1 -> Display27/1
  Fourier11/2 -> Display28/1
  Fourier15/2 -> Display53/1
  Demux4/3 -> Fourier12/1
  [Uph] -> Scope9/1, Demux4/1
  Demux4/4 -> Fourier13/1
  Fourier14/2 -> Display39/1
  Demux4/2 -> Fourier11/1
  Fourier12/2 -> Display30/1
  Fourier13/1 -> Display32/1
  Fourier14/1 -> Display38/1
  Fourier13/2 -> Display34/1
  Demux4/6 -> Fourier15/1
  Fourier24/2 -> Display62/1
  Fourier23/2 -> Display60/1
  Fourier24/1 -> Display61/1
  Fourier22/1 -> Display57/1
  Fourier22/2 -> Display58/1
  Fourier21/2 -> Display55/1
  Fourier25/2 -> Display65/1
  Fourier26/2 -> Display67/1
  Fourier26/1 -> Display66/1
  Fourier23/1 -> Display59/1
  [If] -> Fourier26/1
  [Ic] -> Fourier23/1
  Fourier25/1 -> Display64/1
  [Ib] -> Fourier22/1
  Fourier21/1 -> Display54/1
  [Ie] -> Fourier25/1
  [Id] -> Fourier24/1
  [Ia] -> Fourier21/1
  Subsystem14/3(|u|1) -> Display72/1
  [Uab] -> Subsystem1/1(In1)
  Subsystem14/1(|u|) -> Display76/1
  Demux5/1 -> Subsystem14/1(In1)
  Demux5/2 -> Subsystem14/2(In2)
  [Ufa] -> Subsystem1/6(In6)
  Demux5/3 -> Subsystem14/3(In3)
  Demux5/4 -> Subsystem14/4(In4)
  Demux5/5 -> Subsystem14/5(In5)
  [Uph] -> Demux5/1
  [Ubc] -> Subsystem1/2(In2)
  [Ia] -> Subsystem2/1(In1)
  [Ie] -> Subsystem2/5(In5)
  [Id] -> Subsystem2/4(In4)
  Subsystem2/2(<u) -> Display21/1
  [If] -> Subsystem2/6(In6)
  Subsystem2/1(|u|) -> Display22/1
  [Ib] -> Subsystem2/2(In2)
  [Ic] -> Subsystem2/3(In3)
  Subsystem14/2(<u) -> Display74/1
  Subsystem14/4(<u1) -> Display73/1
  Subsystem1/4(<u1) -> Display8/1
  [Ude] -> Subsystem1/4(In4)
  [Ucd] -> Subsystem1/3(In3)
  Subsystem1/2(<u) -> Display68/1
  [Uef] -> Subsystem1/5(In5)
  Subsystem1/3(|u|1) -> Display7/1
  Demux5/6 -> Subsystem14/6(In6)
  [Ude] -> Fourier18/1
  [Ufa] -> Fourier20/1
  [Uab] -> Fourier9/1
  [Uef] -> Fourier19/1
  Fourier20/2 -> Gain22/1, Display88/1
  Fourier17/1 -> Display81/1, Magnitude-Angle to Complex11/1
  Fourier16/1 -> Magnitude-Angle to Complex10/1, Display79/1
  Fourier19/1 -> Magnitude-Angle to Complex13/1, Display85/1
  Fourier20/1 -> Magnitude-Angle to Complex14/1, Display87/1
  Fourier19/2 -> Gain21/1, Display86/1
  Fourier18/1 -> Display83/1, Magnitude-Angle to Complex12/1
  [Ucd] -> Fourier17/1
  [Ubc] -> Fourier16/1
  Fourier9/2 -> Gain16/1, Display78/1
  Fourier17/2 -> Gain19/1, Display82/1
  Fourier18/2 -> Display84/1, Gain20/1
  Fourier16/2 -> Gain17/1, Display80/1
  Demux4/1 -> Fourier2/1
  [Ip] -> Subsystem15/1(In1)
  [In] -> Subsystem15/2(In2)
  [I0] -> Subsystem15/3(In3)
  Subsystem15/1(Out1) -> Display1/1
  Subsystem15/2(Out2) -> Display89/1
  [Ie] -> Mux7/3
  [Ia] -> Mux7/1
  [Ic] -> Mux7/2
  Mux7/1 -> abc to Alpha-Beta-Zero/1
  abc to Alpha-Beta-Zero/1 -> Scope8/1, Demux/1
  Demux/1 -> Fourier27/1
  Fourier27/2 -> Display97/1, Gain4/1
  Gain4/1 -> Magnitude-Angle to Complex6/2
  Fourier27/1 -> Display96/1, Magnitude-Angle to Complex6/1
  Magnitude-Angle to Complex6/1 -> Display90/1
  Magnitude-Angle to Complex7/1 -> Display91/1
  Fourier28/1 -> Display93/1, Magnitude-Angle to Complex7/1
  Demux/2 -> Fourier28/1
  Gain5/1 -> Magnitude-Angle to Complex7/2
  Fourier28/2 -> Display94/1, Gain5/1
  Fourier29/2 -> Gain7/1
  Gain7/1 -> Magnitude-Angle to Complex9/2
  Magnitude-Angle to Complex9/1 -> Display92/1
  Fourier29/1 -> Magnitude-Angle to Complex9/1
  Demux/3 -> Fourier29/1
  Demux6/2 -> Divide/1
  Demux6/1 -> Divide/2
  Divide/1 -> Display100/1
  Subsystem1/1(|u|) -> Demux6/1, Display69/1
  Subsystem16/2(Out2) -> Display101/1
  [Ufa] -> Subsystem16/6(In6)
  [Uab] -> Subsystem16/1(In1)
  [Ude] -> Subsystem16/4(In4)
  Subsystem16/1(Out1) -> Display112/1
  [Ubc] -> Subsystem16/2(In2)
  [Ucd] -> Subsystem16/3(In3)
  [Uef] -> Subsystem16/5(In5)
  Magnitude-Angle to Complex8/1 -> Display95/1
  Fourier9/1 -> Magnitude-Angle to Complex8/1, Display77/1
  Gain16/1 -> Magnitude-Angle to Complex8/2
  Magnitude-Angle to Complex10/1 -> Display98/1
  Gain17/1 -> Magnitude-Angle to Complex10/2
  Gain19/1 -> Magnitude-Angle to Complex11/2
  Magnitude-Angle to Complex11/1 -> Display99/1
  Gain20/1 -> Magnitude-Angle to Complex12/2
  Magnitude-Angle to Complex12/1 -> Display102/1
  Gain21/1 -> Magnitude-Angle to Complex13/2
  Magnitude-Angle to Complex13/1 -> Display103/1
  Magnitude-Angle to Complex14/1 -> Display104/1
  Gain22/1 -> Magnitude-Angle to Complex14/2
  [Uab] -> Subsystem17/1(In6)
  [Ubc] -> Subsystem17/2(In1)
  [Ucd] -> Subsystem17/3(In2)
  [Ude] -> Subsystem17/4(In3)
  [Uef] -> Subsystem17/5(In4)
  [Ufa] -> Subsystem17/6(In5)
  Subsystem17/1(Out1) -> Scope10/1
  Subsystem17/2(Out2) -> Scope10/2
  Subsystem18/2(Out2) -> Scope11/2
  Subsystem18/1(Out1) -> Scope11/1
  [Ia] -> Subsystem18/1(In6)
  [Ib] -> Subsystem18/2(In1)
  [Ic] -> Subsystem18/3(In2)
  [Id] -> Subsystem18/4(In3)
  [Ie] -> Subsystem18/5(In4)
  [If] -> Subsystem18/6(In5)
  [Uab] -> Subsystem19/1(In1)
  [Ubc] -> Subsystem19/2(In2)
  [Ucd] -> Subsystem19/3(In3)
  [Ude] -> Subsystem19/4(In4)
  [Uef] -> Subsystem19/5(In5)
  [Ufa] -> Subsystem19/6(In6)
  Subsystem19/1(|u|) -> Display12/1
  Subsystem19/2(<u) -> Display16/1
  Subsystem20/2(<u) -> Display106/1
  Subsystem20/1(|u|) -> Display105/1
  [Uac] -> Subsystem20/1(In1)
  [Ubd] -> Subsystem20/2(In2)
  [Ufb] -> Subsystem20/6(In6)
  [Uea] -> Subsystem20/5(In5)
  [Udf] -> Subsystem20/4(In4)
  [Uce] -> Subsystem20/3(In3)
  [Uph] -> Demux7/1
  Subsystem21/2(<u) -> Display108/1
  Subsystem21/1(|u|) -> Display107/1
  Demux7/1 -> Subsystem21/1(In1)
  Demux7/2 -> Subsystem21/2(In2)
  Demux7/4 -> Subsystem21/4(In4)
  Demux7/3 -> Subsystem21/3(In3)
  Demux7/5 -> Subsystem21/5(In5)
  Demux7/6 -> Subsystem21/6(In6)
  connections:
  Current Measurement/LConn1 -- AC Voltage Source/RConn1
  Controlled Current Source3/RConn1 -- Voltage Measurement/LConn2 -- Series RLC Branch/RConn1 -- Controlled Current Source/RConn1 -- Voltage Measurement6/LConn2 -- Controlled Current Source1/RConn1 -- Voltage Measurement1/LConn2 -- Series RLC Branch1/RConn1 -- Series RLC Branch2/RConn1 -- Voltage Measurement2/LConn2 -- Controlled Current Source2/RConn1 -- Voltage Measurement4/LConn2 -- Series RLC Branch4/RConn1 -- Controlled Current Source4/RConn1 -- Controlled Current Source5/RConn1 -- Series RLC Branch5/RConn1 -- Voltage Measurement5/LConn2 -- Series RLC Branch3/RConn1 -- Voltage Measurement3/LConn2
  AC Voltage Source1/RConn1 -- Current Measurement1/LConn1
  Voltage Measurement5/LConn1 -- Voltage Measurement12/LConn2 -- Current Measurement5/RConn1 -- Controlled Current Source5/LConn1 -- Series RLC Branch5/LConn1
  Controlled Current Source4/LConn1 -- Current Measurement4/RConn1 -- Voltage Measurement11/LConn2 -- Voltage Measurement4/LConn1 -- Series RLC Branch4/LConn1
  Current Measurement2/LConn1 -- AC Voltage Source2/RConn1
  AC Voltage Source3/RConn1 -- Current Measurement3/LConn1
  AC Voltage Source5/RConn1 -- Current Measurement5/LConn1
  AC Voltage Source4/RConn1 -- Current Measurement4/LConn1
  Series RLC Branch/LConn1 -- Current Measurement/RConn1 -- Voltage Measurement8/LConn2 -- Controlled Current Source/LConn1 -- Voltage Measurement/LConn1
  Voltage Measurement12/LConn1 -- AC Voltage Source5/LConn1 -- Voltage Measurement10/LConn1 -- AC Voltage Source3/LConn1 -- Voltage Measurement7/LConn1 -- AC Voltage Source2/LConn1 -- Voltage Measurement6/LConn1 -- Voltage Measurement8/LConn1 -- AC Voltage Source/LConn1 -- Voltage Measurement9/LConn1 -- AC Voltage Source1/LConn1 -- Voltage Measurement11/LConn1 -- AC Voltage Source4/LConn1
  Controlled Current Source1/LConn1 -- Current Measurement1/RConn1 -- Voltage Measurement9/LConn2 -- Voltage Measurement1/LConn1 -- Series RLC Branch1/LConn1
  Controlled Current Source2/LConn1 -- Current Measurement2/RConn1 -- Voltage Measurement7/LConn2 -- Voltage Measurement2/LConn1 -- Series RLC Branch2/LConn1
  Voltage Measurement10/LConn2 -- Controlled Current Source3/LConn1 -- Voltage Measurement3/LConn1 -- Series RLC Branch3/LConn1 -- Current Measurement3/RConn1

== system MI6FS_HE_6PhS/RMS VALUES ==
  U : Inport
  I : Inport  Port=2
  Demux : Demux  Outputs=6
      settings: DisplayOption=none
  Demux1 : Demux  Outputs=6
  Divide : Product  Inputs=*/
  Gain1 : Gain  Gain=6
  Gain2 : Gain  Gain=6
  Gain3 : Gain  Gain=6
  Power2 : spsPowerLib/Power  Freq=50  Vinit=[0, 0]  Iinit=[0, 0]  Ts=Ts
  Product : Product
  RMS Measurement : eeRmsMeasurement/RMS Measurement  LabelModeActiveChoice=Total  F=50  SpecifyHarmonics=off  K=[0 1 2]  Ts=0
  RMS Measurement1 : eeRmsMeasurement/RMS Measurement  LabelModeActiveChoice=Total  F=50  SpecifyHarmonics=off  K=[0 1 2]  Ts=Ts
  U1 : Outport  VectorParamsAs1DForOutWhenUnconnected=off
  I1 : Outport  Port=2  VectorParamsAs1DForOutWhenUnconnected=off
  P : Outport  Port=3  VectorParamsAs1DForOutWhenUnconnected=off
  Q : Outport  Port=4  VectorParamsAs1DForOutWhenUnconnected=off
  S : Outport  Port=5  VectorParamsAs1DForOutWhenUnconnected=off
  FP : Outport  Port=6  VectorParamsAs1DForOutWhenUnconnected=off
  wires:
  Demux1/1 -> Power2/1, RMS Measurement1/1
  Divide/1 -> FP/1
  Gain1/1 -> S/1, Divide/2
  Demux/1 -> RMS Measurement/1, Power2/2
  RMS Measurement/1 -> I1/1, Product/2
  I/1 -> Demux/1
  Product/1 -> Gain1/1
  RMS Measurement1/1 -> Product/1, U1/1
  Power2/1 -> Gain3/1
  Power2/2 -> Gain2/1
  U/1 -> Demux1/1
  Gain2/1 -> Q/1
  Gain3/1 -> P/1, Divide/1

== system MI6FS_HE_6PhS/Motor System/MECHANICAL SYSTEM ==
  I_s : Inport
  I_r : Inport  Port=2
  TLoad : Inport  Port=3
  Add : Sum
  Add2 : Sum
  Constant : Constant  Value=Lsr
  Constant1 : Constant  Value=Tav
  Cos : Trigonometry
  Discrete-Time Integrator : DiscreteIntegrator  IntegratorMethod=Integration: Trapezoidal  SampleTime=Ts  ICPrevOutput=DiscIntNeverNeededParam  ICPrevScaledInput=DiscIntNeverNeededParam
  Discrete-Time Integrator1 : DiscreteIntegrator  IntegratorMethod=Integration: Trapezoidal  SampleTime=Ts  ICPrevOutput=DiscIntNeverNeededParam  ICPrevScaledInput=DiscIntNeverNeededParam
  Discrete-Time Integrator2 : DiscreteIntegrator  IntegratorMethod=Integration: Trapezoidal  SampleTime=Ts  ICPrevOutput=DiscIntNeverNeededParam  ICPrevScaledInput=DiscIntNeverNeededParam
  Gain1 : Gain  Gain=1/J
  Gain2 : Gain  Gain=p
  Gain3 : Gain  Gain=60/(2*pi)
  Gain4 : Gain  Gain=Lto
  Gain5 : Gain  Gain=-Msr  Multiplication=Matrix(K*u)
  Gain6 : Gain  Gain=p  Multiplication=Matrix(K*u)
  Product : Product
  Product1 : Product  Multiplication=Matrix(*)
  Product2 : Product  Multiplication=Matrix(*)
  Reshape : Reshape  OutputDimensionality=Customize  OutputDimensions=1
  Reshape1 : Reshape  OutputDimensionality=Customize  OutputDimensions=1
  Sin : Trigonometry
  Subtract1 : Sum  Inputs=+--
  Transpose : Math  Operator=transpose  SignedPower=on
  Unit Delay2 : UnitDelay  SampleTime=Ts  HasFrameUpgradeWarning=on
  We [rads/s] : Outport  VectorParamsAs1DForOutWhenUnconnected=off
  Tem [Nm] : Outport  Port=2  VectorParamsAs1DForOutWhenUnconnected=off
  n [rpm] : Outport  Port=3  VectorParamsAs1DForOutWhenUnconnected=off
  "Teta_R [rad] " : Outport  Port=4  VectorParamsAs1DForOutWhenUnconnected=off
  wires:
  Subtract1/1 -> Gain1/1  "Tem-TL"
  Gain1/1 -> Discrete-Time Integrator1/1  "d/dt Wm"
  I_s/1 -> Transpose/1
  Discrete-Time Integrator/1 -> Unit Delay2/1, "Teta_R [rad] "/1  "Teta R"
  Add/1 -> Sin/1
  I_r/1 -> Product1/2
  Product2/1 -> Subtract1/1, Reshape/1  "Tem"
  Gain3/1 -> Reshape1/1
  Transpose/1 -> Gain6/1
  Discrete-Time Integrator1/1 -> Gain2/1, Gain3/1, Discrete-Time Integrator2/1
  Gain6/1 -> Product2/1
  Product1/1 -> Product2/2
  Constant/1 -> Add/1
  Sin/1 -> Gain5/1
  Gain5/1 -> Product1/1
  Constant1/1 -> Subtract1/3
  Reshape/1 -> Tem [Nm]/1
  Reshape1/1 -> n [rpm]/1
  Gain2/1 -> Discrete-Time Integrator/1, We [rads/s]/1
  Unit Delay2/1 -> Add/2
  Discrete-Time Integrator2/1 -> Cos/1  "Teta R"
  Cos/1 -> Product/2
  Gain4/1 -> Product/1
  Add2/1 -> Subtract1/2
  Product/1 -> Add2/2
  TLoad/1 -> Gain4/1, Add2/1

== system MI6FS_HE_6PhS/Motor System/MOTOR SYSTEM EQUATIONS  ==
  We : Inport
  Us : Inport  Port=2
  Teta_R : Inport  Port=3
  ROTOR SYSTEM : Subsystem
  STATOR SYSTEM : Subsystem
  I_stator : Outport  VectorParamsAs1DForOutWhenUnconnected=off
  "I_rotor " : Outport  Port=2  VectorParamsAs1DForOutWhenUnconnected=off
  wires:
  STATOR SYSTEM/2(d/dt I_s) -> ROTOR SYSTEM/2(d/dt I_s)
  ROTOR SYSTEM/2(d/dt I_r) -> STATOR SYSTEM/3(d/dt I_r)
  Us/1 -> STATOR SYSTEM/1(Us-6)
  Teta_R/1 -> ROTOR SYSTEM/3(Teta_R), STATOR SYSTEM/4(Teta_R)
  We/1 -> ROTOR SYSTEM/4(We), STATOR SYSTEM/5(We)
  STATOR SYSTEM/1(I_s) -> ROTOR SYSTEM/1(I_s), I_stator/1
  ROTOR SYSTEM/1(I_r) -> STATOR SYSTEM/2(I_r), "I_rotor "/1

== system MI6FS_HE_6PhS/Phase System/Subsystem ==
  Up : Inport
  Un : Inport  Port=2
  U0 : Inport  Port=3
  Ip : Inport  Port=4
  In : Inport  Port=5
  I0 : Inport  Port=6
  Create 3x3 Matrix : sharedutil/Create 3x3 Matrix  aMode=aMode
  Divide{1..9} (9 alike) : Product  Inputs=*/
  Z : Outport
  wires:
  Up/1 -> [Up]
  Un/1 -> [Un]
  U0/1 -> [U0]
  Ip/1 -> [Ip]
  In/1 -> [In]
  I0/1 -> [I0]
  [Up] -> Divide2/1
  [Ip] -> Divide2/2
  [In] -> Divide1/2
  [Up] -> Divide1/1
  [Up] -> Divide3/1
  [I0] -> Divide3/2
  [Un] -> Divide4/1
  [Un] -> Divide5/1
  [In] -> Divide5/2
  [I0] -> Divide6/2
  [Un] -> Divide6/1
  [U0] -> Divide7/1
  [Ip] -> Divide7/2
  [In] -> Divide8/2
  [U0] -> Divide8/1
  [I0] -> Divide9/2
  [U0] -> Divide9/1
  Divide2/1 -> Create 3x3 Matrix/1
  Divide5/1 -> Create 3x3 Matrix/5
  [Ip] -> Divide4/2
  Divide9/1 -> Create 3x3 Matrix/9
  Create 3x3 Matrix/1 -> Z/1
  Divide1/1 -> Create 3x3 Matrix/2
  Divide3/1 -> Create 3x3 Matrix/3
  Divide4/1 -> Create 3x3 Matrix/4
  Divide6/1 -> Create 3x3 Matrix/6
  Divide7/1 -> Create 3x3 Matrix/7
  Divide8/1 -> Create 3x3 Matrix/8

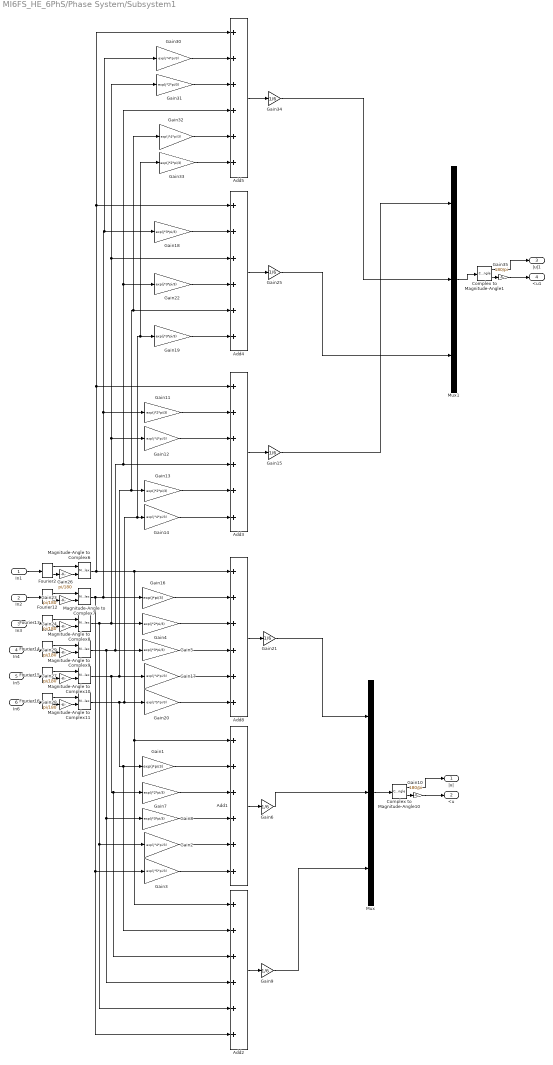
== system MI6FS_HE_6PhS/Phase System/Subsystem1 ==
  In1 : Inport
  In2 : Inport  Port=2
  In3 : Inport  Port=3
  In4 : Inport  Port=4
  In5 : Inport  Port=5
  In6 : Inport  Port=6
  Add{1..5,8} (6 alike) : Sum  Inputs=++++++
  Complex to Magnitude-Angle1 : ComplexToMagnitudeAngle
  Complex to Magnitude-Angle10 : ComplexToMagnitudeAngle
  Fourier{2,12..16} (6 alike) : spsFourierLib/Fourier  Freq=50  n=1  InInit=[0, 0]  Ts=Ts
  Gain1 : Gain  Gain=exp(j*pi/3)
  Gain10 : Gain  Gain=180/pi
  Gain{4,7,11,13,31,33} (6 alike) : Gain  Gain=exp(j*2*pi/3)
  Gain{2,12,14,17,30,32} (6 alike) : Gain  Gain=exp(j*4*pi/3)
  Gain{6,9,15,21,25,34} (6 alike) : Gain  Gain=1/6
  Gain16 : Gain  Gain=exp(j*pi/3)
  Gain{5,8,18..19,22} (5 alike) : Gain  Gain=exp(j*3*pi/3)
  Gain20 : Gain  Gain=exp(j*5*pi/3)
  Gain{23..24,26..29} (6 alike) : Gain  Gain=pi/180
  Gain3 : Gain  Gain=exp(j*5*pi/3)
  Gain35 : Gain  Gain=180/pi
  Magnitude-Angle to Complex{6..11} (6 alike) : MagnitudeAngleToComplex
  Mux : Mux  Inputs=3
  Mux1 : Mux  Inputs=3
  |u| : Outport
  <u : Outport  Port=2
  |u|1 : Outport  Port=3
  <u1 : Outport  Port=4
  wires:
  Gain16/1 -> Add8/2
  Fourier14/2 -> Gain29/1
  Fourier12/2 -> Gain23/1
  Gain27/1 -> Magnitude-Angle to Complex10/2
  Fourier2/2 -> Gain26/1
  Fourier14/1 -> Magnitude-Angle to Complex9/1
  In6/1 -> Fourier16/1
  Magnitude-Angle to Complex7/1 -> Add2/6, Gain3/1, Gain30/1, Gain18/1, Gain11/1, Gain16/1
  Gain28/1 -> Magnitude-Angle to Complex11/2
  In4/1 -> Fourier14/1
  Fourier16/1 -> Magnitude-Angle to Complex11/1
  Fourier2/1 -> Magnitude-Angle to Complex6/1
  Gain4/1 -> Add8/3
  Gain5/1 -> Add8/4
  Magnitude-Angle to Complex10/1 -> Add2/3, Gain7/1, Gain13/1, Gain32/1, Add4/5, Gain17/1
  Magnitude-Angle to Complex9/1 -> Add2/4, Gain8/1, Add5/4, Gain22/1, Add3/4, Gain5/1
  Fourier13/2 -> Gain24/1
  Gain29/1 -> Magnitude-Angle to Complex9/2
  Gain17/1 -> Add8/5
  Gain20/1 -> Add8/6
  In1/1 -> Fourier2/1
  In3/1 -> Fourier13/1
  Fourier16/2 -> Gain28/1
  Fourier15/2 -> Gain27/1
  Fourier15/1 -> Magnitude-Angle to Complex10/1
  Gain23/1 -> Magnitude-Angle to Complex7/2
  Gain24/1 -> Magnitude-Angle to Complex8/2
  Gain26/1 -> Magnitude-Angle to Complex6/2
  Fourier13/1 -> Magnitude-Angle to Complex8/1
  Fourier12/1 -> Magnitude-Angle to Complex7/1
  Add8/1 -> Gain21/1
  Magnitude-Angle to Complex8/1 -> Add2/5, Gain2/1, Gain31/1, Add4/3, Gain12/1, Gain4/1
  In5/1 -> Fourier15/1
  In2/1 -> Fourier12/1
  Gain3/1 -> Add1/6
  Gain8/1 -> Add1/4
  Gain7/1 -> Add1/3
  Gain2/1 -> Add1/5
  Add1/1 -> Gain6/1
  Gain1/1 -> Add1/2
  Magnitude-Angle to Complex6/1 -> Add5/1, Add4/1, Add3/1, Add2/1, Add1/1, Add8/1
  Gain6/1 -> Mux/2
  Add2/1 -> Gain9/1
  Complex to Magnitude-Angle10/2 -> Gain10/1
  Mux/1 -> Complex to Magnitude-Angle10/1
  Gain10/1 -> <u/1
  Complex to Magnitude-Angle10/1 -> |u|/1
  Gain11/1 -> Add3/2
  Gain12/1 -> Add3/3
  Gain13/1 -> Add3/5
  Gain14/1 -> Add3/6
  Add3/1 -> Gain15/1
  Gain18/1 -> Add4/2
  Gain22/1 -> Add4/4
  Gain19/1 -> Add4/6
  Add4/1 -> Gain25/1
  Gain30/1 -> Add5/2
  Gain31/1 -> Add5/3
  Gain32/1 -> Add5/5
  Gain33/1 -> Add5/6
  Magnitude-Angle to Complex11/1 -> Add2/2, Gain1/1, Gain19/1, Gain33/1, Gain14/1, Gain20/1
  Add5/1 -> Gain34/1
  Complex to Magnitude-Angle1/1 -> |u|1/1
  Gain35/1 -> <u1/1
  Complex to Magnitude-Angle1/2 -> Gain35/1
  Mux1/1 -> Complex to Magnitude-Angle1/1
  Gain15/1 -> Mux1/1
  Gain34/1 -> Mux1/2
  Gain25/1 -> Mux1/3
  Gain21/1 -> Mux/1
  Gain9/1 -> Mux/3

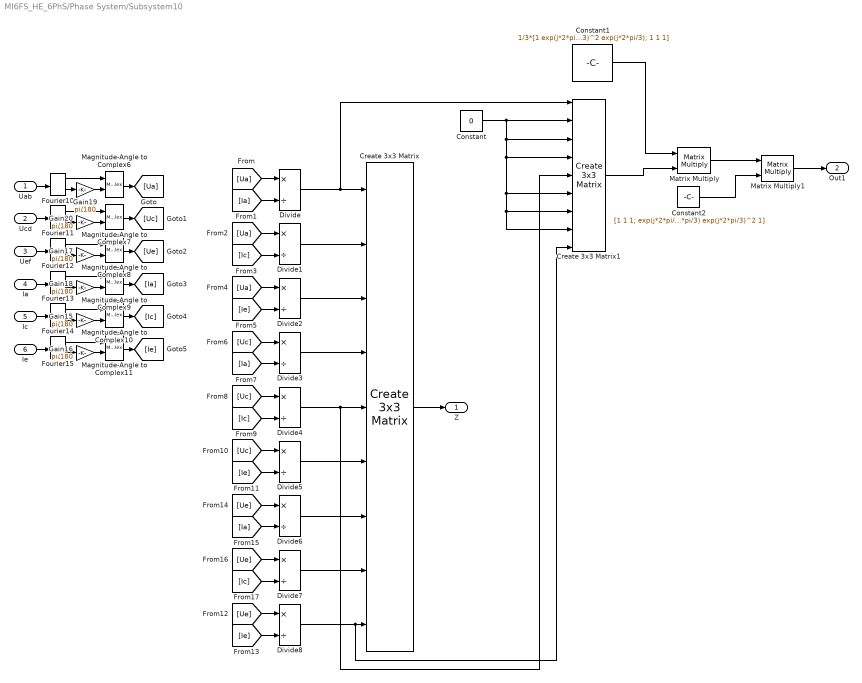
== system MI6FS_HE_6PhS/Phase System/Subsystem10 ==
  Uab : Inport
  Ucd : Inport  Port=2
  Uef : Inport  Port=3
  Ia : Inport  Port=4
  Ic : Inport  Port=5
  Ie : Inport  Port=6
  Constant : Constant  Value=0
  Constant1 : Constant  Value=1/3*[1 exp(j*2*pi/3) exp(j*2*pi/3)^2; 1 exp(j*2*pi/3)^2 exp(j*2*pi/3); 1 1 1]
  Constant2 : Constant  Value=[1 1 1; exp(j*2*pi/3)^2 exp(j*2*pi/3) 1; exp(j*2*pi/3) exp(j*2*pi/3)^2 1]
  Create 3x3 Matrix : sharedutil/Create 3x3 Matrix  aMode=aMode
  Create 3x3 Matrix1 : sharedutil/Create 3x3 Matrix  aMode=aMode
  Divide{,1..8} (9 alike) : Product  Inputs=*/
  Fourier{10..15} (6 alike) : spsFourierLib/Fourier  Freq=50  n=1  InInit=[0, 0]  Ts=Ts
  Gain{15..20} (6 alike) : Gain  Gain=pi/180
  Magnitude-Angle to Complex{6..11} (6 alike) : MagnitudeAngleToComplex
  Matrix Multiply : Product  Multiplication=Matrix(*)
  Matrix Multiply1 : Product  Multiplication=Matrix(*)
  Z : Outport
  Out1 : Outport  Port=2
  wires:
  Gain19/1 -> Magnitude-Angle to Complex6/2
  Ie/1 -> Fourier15/1
  Fourier10/2 -> Gain19/1
  Gain15/1 -> Magnitude-Angle to Complex10/2
  Fourier10/1 -> Magnitude-Angle to Complex6/1
  Fourier13/2 -> Gain18/1
  Gain17/1 -> Magnitude-Angle to Complex8/2
  Fourier11/2 -> Gain20/1
  Fourier15/2 -> Gain16/1
  Gain18/1 -> Magnitude-Angle to Complex9/2
  Fourier14/1 -> Magnitude-Angle to Complex10/1
  Fourier14/2 -> Gain15/1
  Fourier12/2 -> Gain17/1
  Fourier12/1 -> Magnitude-Angle to Complex8/1
  Ic/1 -> Fourier14/1
  Gain20/1 -> Magnitude-Angle to Complex7/2
  Fourier15/1 -> Magnitude-Angle to Complex11/1
  Fourier13/1 -> Magnitude-Angle to Complex9/1
  Fourier11/1 -> Magnitude-Angle to Complex7/1
  Gain16/1 -> Magnitude-Angle to Complex11/2
  Uab/1 -> Fourier10/1
  Ia/1 -> Fourier13/1
  Uef/1 -> Fourier12/1
  Ucd/1 -> Fourier11/1
  Magnitude-Angle to Complex6/1 -> [Ua]
  Magnitude-Angle to Complex7/1 -> [Uc]
  Magnitude-Angle to Complex8/1 -> [Ue]
  Magnitude-Angle to Complex9/1 -> [Ia]
  Magnitude-Angle to Complex10/1 -> [Ic]
  Magnitude-Angle to Complex11/1 -> [Ie]
  [Ua] -> Divide/1
  [Ia] -> Divide/2
  [Ua] -> Divide1/1
  [Ic] -> Divide1/2
  [Ua] -> Divide2/1
  [Ie] -> Divide2/2
  Divide1/1 -> Create 3x3 Matrix/2
  Divide5/1 -> Create 3x3 Matrix/6
  [Ie] -> Divide5/2
  [Uc] -> Divide5/1
  [Ic] -> Divide4/2
  [Uc] -> Divide4/1
  Divide3/1 -> Create 3x3 Matrix/4
  [Ia] -> Divide3/2
  [Uc] -> Divide3/1
  [Ue] -> Divide7/1
  [Ic] -> Divide7/2
  [Ia] -> Divide6/2
  Divide6/1 -> Create 3x3 Matrix/7
  [Ie] -> Divide8/2
  [Ue] -> Divide8/1
  [Ue] -> Divide6/1
  Divide7/1 -> Create 3x3 Matrix/8
  Divide2/1 -> Create 3x3 Matrix/3
  Create 3x3 Matrix/1 -> Z/1
  Constant1/1 -> Matrix Multiply/1
  Constant/1 -> Create 3x3 Matrix1/8, Create 3x3 Matrix1/7, Create 3x3 Matrix1/6, Create 3x3 Matrix1/4, Create 3x3 Matrix1/3, Create 3x3 Matrix1/2
  Create 3x3 Matrix1/1 -> Matrix Multiply/2
  Divide8/1 -> Create 3x3 Matrix1/9, Create 3x3 Matrix/9
  Matrix Multiply1/1 -> Out1/1
  Matrix Multiply/1 -> Matrix Multiply1/1
  Divide/1 -> Create 3x3 Matrix1/1, Create 3x3 Matrix/1
  Constant2/1 -> Matrix Multiply1/2
  Divide4/1 -> Create 3x3 Matrix1/5, Create 3x3 Matrix/5

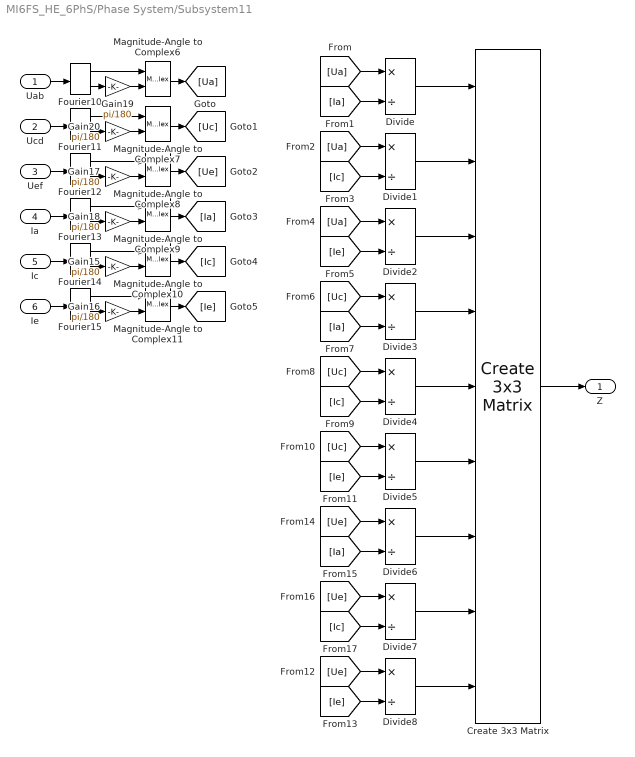
== system MI6FS_HE_6PhS/Phase System/Subsystem11 ==
  Uab : Inport
  Ucd : Inport  Port=2
  Uef : Inport  Port=3
  Ia : Inport  Port=4
  Ic : Inport  Port=5
  Ie : Inport  Port=6
  Create 3x3 Matrix : sharedutil/Create 3x3 Matrix  aMode=aMode
  Divide{,1..8} (9 alike) : Product  Inputs=*/
  Fourier{10..15} (6 alike) : spsFourierLib/Fourier  Freq=50  n=1  InInit=[0, 0]  Ts=Ts
  Gain{15..20} (6 alike) : Gain  Gain=pi/180
  Magnitude-Angle to Complex{6..11} (6 alike) : MagnitudeAngleToComplex
  Z : Outport
  wires:
  Gain19/1 -> Magnitude-Angle to Complex6/2
  Ie/1 -> Fourier15/1
  Fourier10/2 -> Gain19/1
  Gain15/1 -> Magnitude-Angle to Complex10/2
  Fourier10/1 -> Magnitude-Angle to Complex6/1
  Fourier13/2 -> Gain18/1
  Gain17/1 -> Magnitude-Angle to Complex8/2
  Fourier11/2 -> Gain20/1
  Fourier15/2 -> Gain16/1
  Gain18/1 -> Magnitude-Angle to Complex9/2
  Fourier14/1 -> Magnitude-Angle to Complex10/1
  Fourier14/2 -> Gain15/1
  Fourier12/2 -> Gain17/1
  Fourier12/1 -> Magnitude-Angle to Complex8/1
  Ic/1 -> Fourier14/1
  Gain20/1 -> Magnitude-Angle to Complex7/2
  Fourier15/1 -> Magnitude-Angle to Complex11/1
  Fourier13/1 -> Magnitude-Angle to Complex9/1
  Fourier11/1 -> Magnitude-Angle to Complex7/1
  Gain16/1 -> Magnitude-Angle to Complex11/2
  Uab/1 -> Fourier10/1
  Ia/1 -> Fourier13/1
  Uef/1 -> Fourier12/1
  Ucd/1 -> Fourier11/1
  Magnitude-Angle to Complex6/1 -> [Ua]
  Magnitude-Angle to Complex7/1 -> [Uc]
  Magnitude-Angle to Complex8/1 -> [Ue]
  Magnitude-Angle to Complex9/1 -> [Ia]
  Magnitude-Angle to Complex10/1 -> [Ic]
  Magnitude-Angle to Complex11/1 -> [Ie]
  [Ua] -> Divide/1
  [Ia] -> Divide/2
  Divide/1 -> Create 3x3 Matrix/1
  [Ua] -> Divide1/1
  [Ic] -> Divide1/2
  [Ua] -> Divide2/1
  [Ie] -> Divide2/2
  Divide1/1 -> Create 3x3 Matrix/2
  Divide5/1 -> Create 3x3 Matrix/6
  Divide4/1 -> Create 3x3 Matrix/5
  [Ie] -> Divide5/2
  [Uc] -> Divide5/1
  [Ic] -> Divide4/2
  [Uc] -> Divide4/1
  Divide3/1 -> Create 3x3 Matrix/4
  [Ia] -> Divide3/2
  [Uc] -> Divide3/1
  [Ue] -> Divide7/1
  Divide8/1 -> Create 3x3 Matrix/9
  [Ic] -> Divide7/2
  [Ia] -> Divide6/2
  Divide6/1 -> Create 3x3 Matrix/7
  [Ie] -> Divide8/2
  [Ue] -> Divide8/1
  [Ue] -> Divide6/1
  Divide7/1 -> Create 3x3 Matrix/8
  Divide2/1 -> Create 3x3 Matrix/3
  Create 3x3 Matrix/1 -> Z/1
